simulink model "storpedo"  (R2020a)
settings: Solver=ode45  StartTime=0.0  StopTime=10  RelTol=1e-3
values from neighbouring files (symbols this model uses):
  k1 = 30    [torpedo.m]
  k2_1 = 1    [torpedo.m]
  k2_2 = 1    [torpedo.m]
  k3 = 5    [torpedo.m]
  v = 10    [car_suspension.m]    (also in main.m = 20; torpedo.m = 40)
  v1 = 40    [torpedo.m]
settings Model: Creator=ACER  LastModifiedBy=ACER

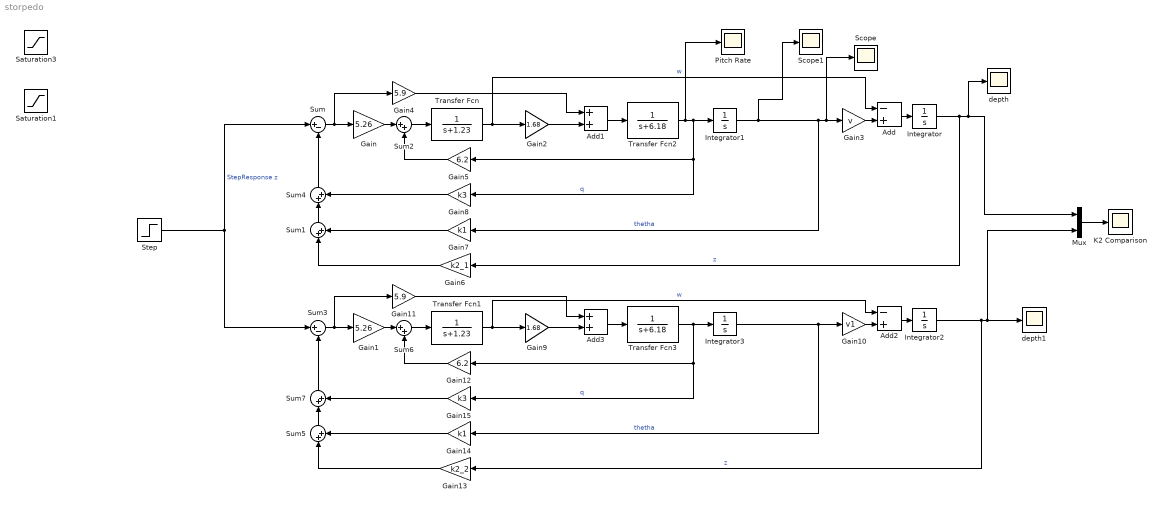
== system storpedo ==
  Add : Sum  Inputs=-+
  Add1 : Sum
  Add2 : Sum  Inputs=-+
  Add3 : Sum
  Gain : Gain  Gain=5.26
  Gain1 : Gain  Gain=5.26
  Gain10 : Gain  Gain=v1
  Gain11 : Gain  Gain=5.9
  Gain12 : Gain  Gain=6.2
  Gain13 : Gain  Gain=k2_2
  Gain14 : Gain  Gain=k1
  Gain15 : Gain  Gain=k3
  Gain2 : Gain  Gain=1.68
  Gain3 : Gain  Gain=v
  Gain4 : Gain  Gain=5.9
  Gain5 : Gain  Gain=6.2
  Gain6 : Gain  Gain=k2_1
  Gain7 : Gain  Gain=k1
  Gain8 : Gain  Gain=k3
  Gain9 : Gain  Gain=1.68
  Integrator{,1..3} (4 alike) : Integrator
  K2 Comparison : Scope
  Mux : Mux  Inputs=2
  "Pitch Rate " : Scope
  Saturation1 : Saturate  UpperLimit=5  LowerLimit=-5
  Saturation3 : Saturate  UpperLimit=5  LowerLimit=-5
  Scope : Scope
  Scope1 : Scope
  Step : Step  SampleTime=0
  Sum : Sum  Inputs=|+-
  Sum{1..2,4..7} (6 alike) : Sum  Inputs=|++
  Sum3 : Sum  Inputs=|+-
  Transfer Fcn : TransferFcn  Denominator=[1 1.23]
  Transfer Fcn1 : TransferFcn  Denominator=[1 1.23]
  Transfer Fcn2 : TransferFcn  Denominator=[1 6.18]
  Transfer Fcn3 : TransferFcn  Denominator=[1 6.18]
  depth : Scope
  depth1 : Scope
  wires:
  Sum/1 -> Gain/1, Gain4/1
  Gain/1 -> Sum2/1
  Sum2/1 -> Transfer Fcn/1
  Transfer Fcn/1 -> Add/1, Gain2/1  "w"
  Gain2/1 -> Add1/2
  Add1/1 -> Transfer Fcn2/1
  Transfer Fcn2/1 -> Integrator1/1, Gain8/1, Gain5/1, "Pitch Rate "/1  "q"
  Gain3/1 -> Add/2
  Gain4/1 -> Add1/1
  Gain5/1 -> Sum2/2
  Add/1 -> Integrator/1
  Integrator/1 -> Mux/1, depth/1, Gain6/1  "z"
  Gain6/1 -> Sum1/1
  Gain7/1 -> Sum1/2
  Sum1/1 -> Sum4/1
  Gain8/1 -> Sum4/2
  Sum4/1 -> Sum/2
  Integrator1/1 -> Gain7/1, Scope/1, Gain3/1, Scope1/1  "thetha"
  Integrator3/1 -> Gain14/1, Gain10/1  "thetha"
  Integrator2/1 -> depth1/1, Mux/2, Gain13/1  "z"
  Sum7/1 -> Sum3/2
  Sum5/1 -> Sum7/1
  Gain15/1 -> Sum7/2
  Gain13/1 -> Sum5/1
  Add2/1 -> Integrator2/1
  Gain9/1 -> Add3/2
  Transfer Fcn3/1 -> Integrator3/1, Gain15/1, Gain12/1  "q"
  Gain1/1 -> Sum6/1
  Gain14/1 -> Sum5/2
  Gain11/1 -> Add3/1
  Gain12/1 -> Sum6/2
  Sum6/1 -> Transfer Fcn1/1
  Sum3/1 -> Gain1/1, Gain11/1
  Add3/1 -> Transfer Fcn3/1
  Gain10/1 -> Add2/2
  Transfer Fcn1/1 -> Gain9/1, Add2/1  "w"
  Step/1 -> Sum3/1, Sum/1  "StepResponse z"
  Mux/1 -> K2 Comparison/1
